simulink model "pos_est_sil"  (R2024a)
settings: Solver=FixedStepAuto  StartTime=0.0  StopTime=600  FixedStep=0.02  RelTol=1e-3
libraries: simulink_extras x3
settings Model: Creator=Zhenkai  LastModifiedBy=Zhenkai
settings DataIOCC: ReturnWorkspaceOutputs=off

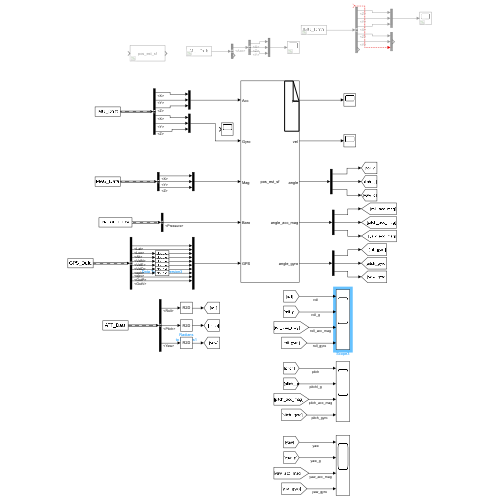
[thumbnail: Simulink's stored preview of the top-level diagram]
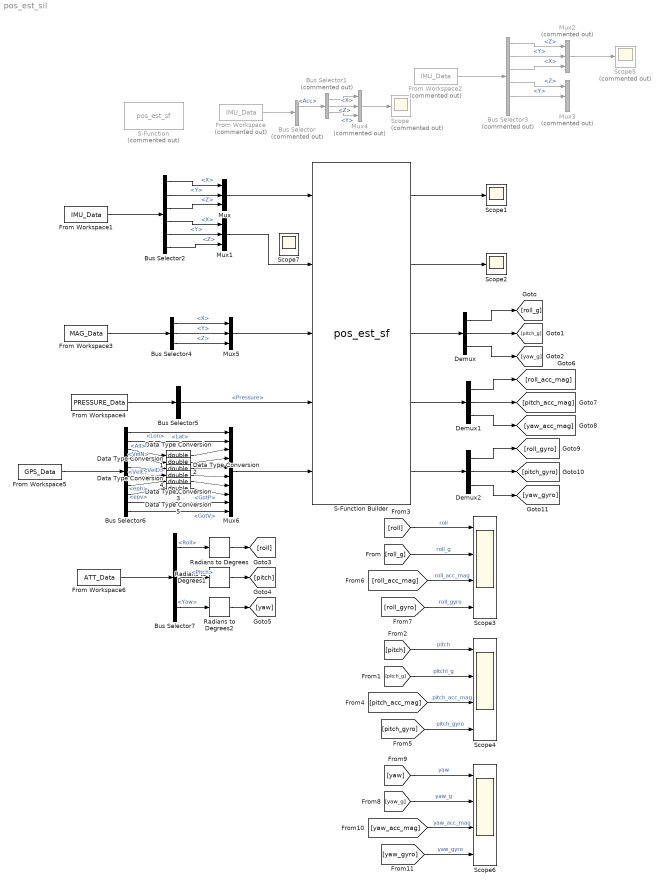
== system pos_est_sil ==
  Bus Selector : BusSelector  Commented=on  OutputSignals=Acc,Gyro
  Bus Selector1 : BusSelector  Commented=on  OutputSignals=X,Z,Y
  Bus Selector2 : BusSelector  OutputSignals=Acc.X,Acc.Y,Acc.Z,Gyro.X,Gyro.Y,Gyro.Z
  Bus Selector3 : BusSelector  Commented=on  OutputSignals=Gyro.Z,Gyro.Y,Gyro.X,Acc.Z,Acc.Y,Acc.X
  Bus Selector4 : BusSelector  OutputSignals=X,Y,Z
  Bus Selector5 : BusSelector  OutputSignals=Pressure
  Bus Selector6 : BusSelector  OutputSignals=Lat,Lon,Alt,VelN,VelE,VelD,eph,epv,GotP,GotV
  Bus Selector7 : BusSelector  OutputSignals=Roll,Pitch,Yaw
  Data Type Conversion{,1..5} (6 alike) : DataTypeConversion  OutDataTypeStr=double  SaturateOnIntegerOverflow=off  RndMeth=Floor
  Demux : Demux  Outputs=3
  Demux1 : Demux  Outputs=3
  Demux2 : Demux  Outputs=3
  From Workspace : FromWorkspace  Commented=on  VariableName=IMU_Data  OutDataTypeStr=Bus: IMU_Bus  Interpolate=off  ZeroCross=off  OutputAfterFinalValue=Holding final value
  From Workspace1 : FromWorkspace  VariableName=IMU_Data  OutDataTypeStr=Bus: IMU_Bus
  From Workspace2 : FromWorkspace  Commented=on  VariableName=IMU_Data  OutDataTypeStr=Bus: IMU_Bus  Interpolate=off
  From Workspace3 : FromWorkspace  VariableName=MAG_Data  OutDataTypeStr=Bus: MAG_Bus
  From Workspace4 : FromWorkspace  VariableName=PRESSURE_Data  OutDataTypeStr=Bus: PRESSURE_Bus
  From Workspace5 : FromWorkspace  VariableName=GPS_Data  OutDataTypeStr=Bus: GPS_Bus
  From Workspace6 : FromWorkspace  VariableName=ATT_Data  OutDataTypeStr=Bus: ATT_Bus
  Mux : Mux  Inputs=3
  Mux1 : Mux  Inputs=3
  Mux2 : Mux  Commented=on  Inputs=3
  Mux3 : Mux  Commented=on  Inputs=3
  Mux4 : Mux  Commented=on  Inputs=3
  Mux5 : Mux  Inputs=3
  Mux6 : Mux  Inputs=10
  Radians to Degrees : simulink_extras/Transformations/Radians to Degrees
  Radians to Degrees1 : simulink_extras/Transformations/Radians to Degrees
  Radians to Degrees2 : simulink_extras/Transformations/Radians to Degrees
  S-Function : S-Function  Commented=on  FunctionName=pos_est_sf  SFunctionDeploymentMode=off  EnableBusSupport=off
  S-Function Builder : S-Function  FunctionName=pos_est_sf  SFunctionModules=pos_est_sf_wrapper.c ringbuff com_data pro_common filter mahony attitude_estimate position_estimate task_integrated_navigation  SFunctionDeploymentMode=off  EnableBusSupport=off  mask(S-Function Builder){}
      mask help: Simulink:masks:SFunctionBuilder_MD
      mask init:
      | val = [[.9  0.75 0.75 1 1 .9 .9 1]',[1 1 0.75 0.75 .9 .9 1 .9]'];try , sys = get_param(gcb,'SfunBuilderFcnName');if isempty(sys), sys = get_param(gcb,'FunctionName'); end,catch, sys = get_param(gcb,'FunctionName'); end
      settings: CopyFcn=set_param(gcbh,'LinkStatus','none')  OpenFcn=sfunctionwizard(gcbh)
      mask Display:
      | plot(val(:,1),val(:,2))
      | disp(sys)
      | port_label('input',1,sprintf('%s', 'Acc'),'interpreter','tex')
      | port_label('input',2,sprintf('%s', 'Gyro'),'interpreter','tex')
      | port_label('input',3,sprintf('%s', 'Mag'),'interpreter','tex')
      | port_label('input',4,sprintf('%s', 'Baro'),'interpreter','tex')
      | port_label('input',5,sprintf('%s', 'GPS'),'interpreter','tex')
      | port_label('output',1,sprintf('%s', 'pos'),'interpreter','tex')
      | port_label('output',2,sprintf('%s', 'vel'),'interpreter','tex')
      | port_label('output',3,sprintf('%s', 'angle'),'interpreter','tex')
      | port_label('output',4,sprintf('%s', 'angle\_acc\_mag'),'interpreter','tex')
      | port_label('output',5,sprintf('%s', 'angle\_gyro'),'interpreter','tex')
  Scope : Scope  Commented=on
  Scope1 : Scope
  Scope2 : Scope
  Scope3 : Scope  NumInputPorts=4
  Scope4 : Scope  NumInputPorts=4
  Scope5 : Scope  Commented=on
  Scope6 : Scope  NumInputPorts=4
  Scope7 : Scope
  wires:
  From Workspace/1 -> Bus Selector/1
  Bus Selector/1 -> Bus Selector1/1  "<Acc>"
  From Workspace1/1 -> Bus Selector2/1
  S-Function Builder/1 -> Scope1/1
  S-Function Builder/2 -> Scope2/1
  Mux/1 -> S-Function Builder/1
  Mux1/1 -> S-Function Builder/2
  Bus Selector3/2 -> Mux2/2  "<Y>"
  Bus Selector3/5 -> Mux3/2  "<Y>"
  Bus Selector3/3 -> Mux2/3  "<X>"
  ? -> Mux3/3
  From Workspace2/1 -> Bus Selector3/1
  Mux2/1 -> Scope5/1
  Bus Selector3/1 -> Mux2/1  "<Z>"
  Bus Selector3/4 -> Mux3/1  "<Z>"
  Bus Selector1/1 -> Mux4/1  "<X>"
  Bus Selector1/2 -> Mux4/2  "<Z>"
  Bus Selector1/3 -> Mux4/3  "<Y>"
  Mux4/1 -> Scope/1
  From Workspace3/1 -> Bus Selector4/1
  Bus Selector4/1 -> Mux5/1  "<X>"
  Bus Selector4/2 -> Mux5/2  "<Y>"
  Bus Selector4/3 -> Mux5/3  "<Z>"
  From Workspace4/1 -> Bus Selector5/1
  From Workspace5/1 -> Bus Selector6/1
  Bus Selector6/1 -> Mux6/1  "<Lat>"
  Bus Selector6/2 -> Mux6/2  "<Lon>"
  Bus Selector6/3 -> Data Type Conversion/1  "<Alt>"
  Bus Selector6/4 -> Data Type Conversion1/1  "<VelN>"
  Bus Selector6/5 -> Data Type Conversion2/1  "<VelE>"
  Bus Selector6/6 -> Data Type Conversion3/1  "<VelD>"
  Bus Selector5/1 -> S-Function Builder/4  "<Pressure>"
  Mux5/1 -> S-Function Builder/3
  Mux6/1 -> S-Function Builder/5
  Bus Selector6/7 -> Data Type Conversion4/1  "<eph>"
  Bus Selector6/8 -> Data Type Conversion5/1  "<epv>"
  Bus Selector6/9 -> Mux6/9  "<GotP>"
  Bus Selector6/10 -> Mux6/10  "<GotV>"
  Bus Selector2/1 -> Mux/1  "<X>"
  Bus Selector2/2 -> Mux/2  "<Y>"
  Bus Selector2/3 -> Mux/3  "<Z>"
  Bus Selector2/4 -> Mux1/1  "<X>"
  Bus Selector2/5 -> Mux1/2  "<Y>"
  Bus Selector2/6 -> Mux1/3  "<Z>"
  From Workspace6/1 -> Bus Selector7/1
  S-Function Builder/3 -> Demux/1
  Demux/1 -> [roll_g]
  Demux/3 -> [yaw_g]
  Demux/2 -> [pitch_g]
  Bus Selector7/1 -> Radians to Degrees/1  "<Roll>"
  Bus Selector7/3 -> Radians to Degrees2/1  "<Yaw>"
  Bus Selector7/2 -> Radians to Degrees1/1  "<Pitch>"
  [roll] -> Scope3/1  "roll"
  [roll_g] -> Scope3/2  "roll_g"
  Radians to Degrees/1 -> [roll]
  Radians to Degrees1/1 -> [pitch]
  Radians to Degrees2/1 -> [yaw]
  Demux1/2 -> [pitch_acc_mag]
  Demux1/3 -> [yaw_acc_mag]
  Demux1/1 -> [roll_acc_mag]
  S-Function Builder/4 -> Demux1/1
  S-Function Builder/5 -> Demux2/1
  Demux2/1 -> [roll_gyro]
  Demux2/3 -> [yaw_gyro]
  Demux2/2 -> [pitch_gyro]
  [roll_acc_mag] -> Scope3/3  "roll_acc_mag"
  [roll_gyro] -> Scope3/4  "roll_gyro"
  [pitch_gyro] -> Scope4/4  "pitch_gyro"
  [pitch_acc_mag] -> Scope4/3  "pitch_acc_mag"
  [pitch_g] -> Scope4/2  "pitchl_g"
  [pitch] -> Scope4/1  "pitch"
  [yaw] -> Scope6/1  "yaw"
  [yaw_g] -> Scope6/2  "yaw_g"
  [yaw_acc_mag] -> Scope6/3  "yaw_acc_mag"
  [yaw_gyro] -> Scope6/4  "yaw_gyro"
  Data Type Conversion/1 -> Mux6/3
  Data Type Conversion1/1 -> Mux6/4
  Data Type Conversion2/1 -> Mux6/5
  Data Type Conversion3/1 -> Mux6/6
  Data Type Conversion4/1 -> Mux6/7
  Data Type Conversion5/1 -> Mux6/8
